simulink model "model_sin_no_disturbance"  (R2019b)
settings: Solver=VariableStepAuto  StartTime=0.0  StopTime=500.0  RelTol=1e-3
libraries: fuzblock x1
settings Model: Creator=rafa  LastModifiedBy=rafa

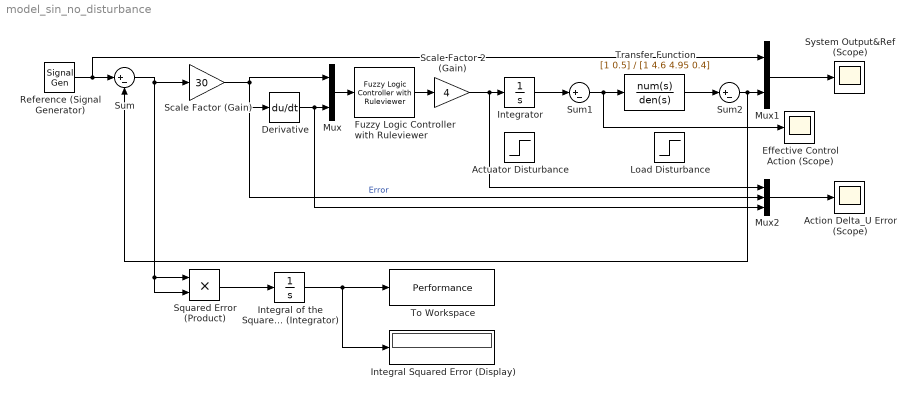
== system model_sin_no_disturbance ==
  Action Delta_U Error (Scope) : Scope
  Actuator Disturbance : Step  Time=100  SampleTime=0
  "Derivative " : Derivative  CoefficientInTFapproximation=Inf
  Effective Control Action (Scope) : Scope
  Fuzzy Logic Controller with Ruleviewer : fuzblock/Fuzzy Logic  Controller  with Ruleviewer  fismatrix=fis  Ts=200
  "Integral Squared Error (Display) " : Display
  Integral of the Squared Error (Integrator) : Integrator
  "Integrator " : Integrator
  Load Disturbance : Step  Time=100  SampleTime=0
  Mux : Mux  Inputs=2
  Mux1 : Mux  Inputs=2
  Mux2 : Mux  Inputs=3
  Reference (Signal Generator) : SignalGenerator  Frequency=0.05  Units=rad/sec
  Scale Factor (Gain) : Gain  Gain=30
  Scale Factor 2 (Gain) : Gain  Gain=4
  Squared Error (Product) : Product
  Sum : Sum  Inputs=|+-
  Sum1 : Sum  Inputs=|+-
  Sum2 : Sum  Inputs=|+-
  System Output&Ref (Scope) : Scope
  "To Workspace " : ToWorkspace  VariableName=Performance  SaveFormat=Timeseries  SampleTime=-1
  "Transfer Function " : TransferFcn  Numerator=[1 0.5]  Denominator=[1 4.6 4.95 0.4]
  wires:
  Reference (Signal Generator)/1 -> Mux1/1, Sum/1
  Sum/1 -> Squared Error (Product)/2, Squared Error (Product)/1, Scale Factor (Gain)/1
  Squared Error (Product)/1 -> Integral of the Squared Error (Integrator)/1
  Integral of the Squared Error (Integrator)/1 -> "Integral Squared Error (Display) "/1, "To Workspace "/1
  Scale Factor (Gain)/1 -> Mux/1, Mux2/2, "Derivative "/1  "Error"
  "Derivative "/1 -> Mux2/3, Mux/2
  Mux/1 -> Fuzzy Logic Controller with Ruleviewer/1
  Fuzzy Logic Controller with Ruleviewer/1 -> Scale Factor 2 (Gain)/1
  Scale Factor 2 (Gain)/1 -> Mux2/1, "Integrator "/1
  "Integrator "/1 -> Sum1/1
  Sum1/1 -> Effective Control Action (Scope)/1, "Transfer Function "/1
  "Transfer Function "/1 -> Sum2/1
  Sum2/1 -> Mux1/2, Sum/2
  Mux1/1 -> System Output&Ref (Scope)/1
  Mux2/1 -> Action Delta_U Error (Scope)/1
